simulink model "Fullsim_MPC"  (R2025b)
settings: Solver=ode4  StartTime=0.0  StopTime=100  FixedStep=0.01  RelTol=1e-3
values from neighbouring files (symbols this model uses):
  psi_op = pi/2    (= 1.57079632679)    [init_linearization.m]
  theta_op = -10*pi/180    (= -0.174532925199)    [init_linearization.m]
  V_mp_op = (K_yy*m_heli*g*cos(theta_op)*l_cm)/(K_yy*K_pp-K_yp*K_py)    [init_linearization.m]
  V_my_op = (K_yp*V_mp_op)/K_yy    [init_linearization.m]
  w_psi_op = 0    [init_linearization.m]
  w_theta_op = 0    [init_linearization.m]
libraries: realtime_pacer_lib x1
settings Model: Creator=bulve  LastModifiedBy=Torstein
settings DebuggingCC: SignalInfNanChecking=error

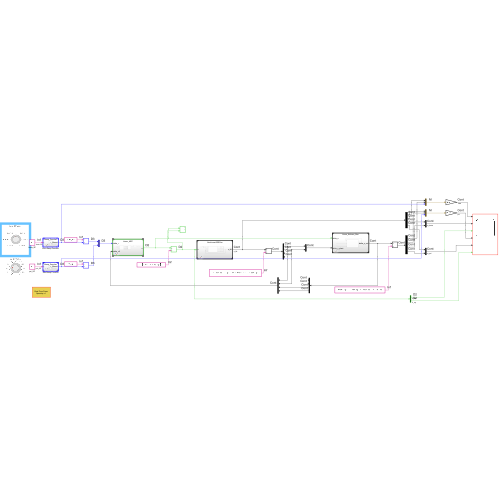
[thumbnail: Simulink's stored preview of the top-level diagram]
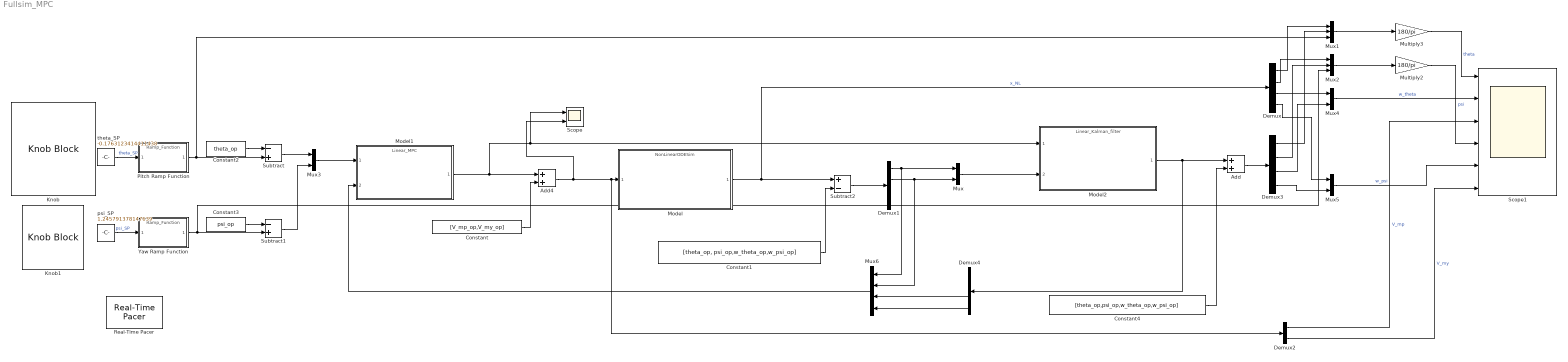
== system Fullsim_MPC ==
  Add : Sum
  Add4 : Sum
  Constant : Constant  Value=[V_mp_op,V_my_op]
  Constant1 : Constant  Value=[theta_op, psi_op,w_theta_op,w_psi_op]
  Constant2 : Constant  Value=theta_op
  Constant3 : Constant  Value=psi_op
  Constant4 : Constant  Value=[theta_op,psi_op,w_theta_op,w_psi_op]
  Demux{,1,3..4} (4 alike) : Demux
  Demux2 : Demux  Outputs=2
  Knob : KnobBlock  ScaleMin=-0.6745  ScaleMax=0.3255
  Knob1 : KnobBlock  ScaleMin=1  ScaleMax=2
  Model : ModelReference  ModelNameDialog=NonLinearODESim.slx  SimulationMode=Normal  ModelReferenceVersion=1.13
  Model1 : ModelReference  ModelNameDialog=Linear_MPC.slx  SimulationMode=Normal  ModelReferenceVersion=1.33
  Model2 : ModelReference  ModelNameDialog=Linear_Kalman_filter.slx  SimulationMode=Normal  ModelReferenceVersion=1.20
  Multiply2 : Gain  Gain=180/pi
  Multiply3 : Gain  Gain=180/pi
  Mux{,3..5} (4 alike) : Mux  Inputs=2
  Mux1 : Mux  Inputs=3
  Mux2 : Mux  Inputs=3
  Mux6 : Mux
  Pitch Ramp Function : ModelReference  ModelNameDialog=Ramp_Function.slx  SimulationMode=Normal  ModelReferenceVersion=1.11
  Real-Time Pacer : realtime_pacer_lib/Real-Time Pacer  simTimePerRealTime=1
      settings: SourceProductName=Real-Time Pacer
  Scope : Scope  NumInputPorts=2
      settings: ActiveDisplayYMinimum=-0.2593542905840886  ActiveDisplayYMaximum=2.3341886152567977
  Scope1 : Scope  NumInputPorts=6
      settings: ActiveDisplayYMinimum=-25.320007216708632  ActiveDisplayYMaximum=0.13277549163516245
  Subtract : Sum  Inputs=-+
  Subtract1 : Sum  Inputs=-+
  Subtract2 : Sum  Inputs=+-
  Yaw Ramp Function : ModelReference  ModelNameDialog=Ramp_Function.slx  SimulationMode=Normal  ModelReferenceVersion=1.11
  psi_SP : Constant  Value=1.245791378147639
  theta_SP : Constant  Value=-0.1763123414411438
  wires:
  psi_SP/1 -> Yaw Ramp Function/1  "psi_SP"
  theta_SP/1 -> Pitch Ramp Function/1  "theta_SP"
  Constant3/1 -> Subtract1/1
  Constant2/1 -> Subtract/1
  Mux3/1 -> Model1/1
  Add4/1 -> Scope/2, Demux2/1, Model/1
  Constant1/1 -> Subtract2/2
  Model2/1 -> Demux4/1, Add/1
  Model1/1 -> Add4/1, Scope/1, Model2/1
  Constant/1 -> Add4/2
  Model/1 -> Subtract2/1, Demux/1  "x_NL"
  Mux2/1 -> Multiply2/1
  Mux1/1 -> Multiply3/1
  Demux/3 -> Mux4/1
  Constant4/1 -> Add/2
  Add/1 -> Demux3/1
  Demux3/3 -> Mux4/2
  Demux/4 -> Mux5/1
  Demux3/4 -> Mux5/2
  Multiply3/1 -> Scope1/1  "theta"
  Subtract/1 -> Mux3/1
  Subtract1/1 -> Mux3/2
  Subtract2/1 -> Demux1/1
  Demux1/1 -> Mux6/1, Mux/1
  Demux1/2 -> Mux6/2, Mux/2
  Mux/1 -> Model2/2
  Demux4/3 -> Mux6/3
  Demux4/4 -> Mux6/4
  Mux6/1 -> Model1/2
  Demux/1 -> Mux1/1
  Demux/2 -> Mux2/1
  Demux3/2 -> Mux2/2
  Demux3/1 -> Mux1/2
  Yaw Ramp Function/1 -> Mux2/3, Subtract1/2
  Pitch Ramp Function/1 -> Subtract/2, Mux1/3
  Multiply2/1 -> Scope1/4  "psi"
  Mux4/1 -> Scope1/2  "w_theta"
  Demux2/1 -> Scope1/3  "V_mp"
  Mux5/1 -> Scope1/5  "w_psi"
  Demux2/2 -> Scope1/6  "V_my"
